simulink model "Q3b_state_space"  (R2025b)
settings: Solver=ode4  StartTime=0.0  StopTime=12.0  FixedStep=0.001  RelTol=1e-3
values from neighbouring files (symbols this model uses):
  A_aug = [A(1,1), A(1,2), 0, 0 ... (first row only)    [ME780_Part3b_Bicycle_DLC.m]
  B_aug = [B ... (first row only)    [ME780_Part3b_Bicycle_DLC.m]
  C_aug = [1,       0,          0, 0 ... (first row only)    [ME780_Part3b_Bicycle_DLC.m]
  D_aug = [0 ... (first row only)    [ME780_Part3b_Bicycle_DLC.m]
settings Model: Creator=r3anjum  LastModifiedBy=r3anjum

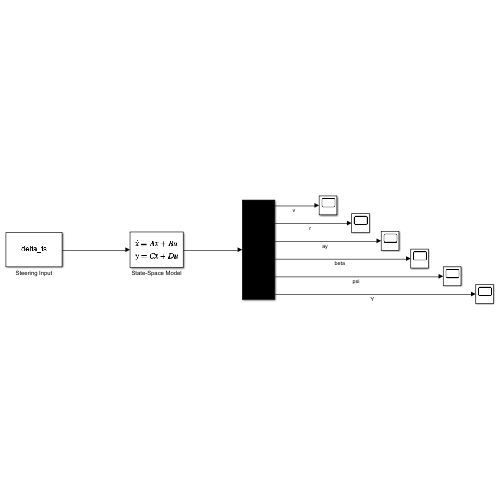
[thumbnail: Simulink's stored preview of the top-level diagram]
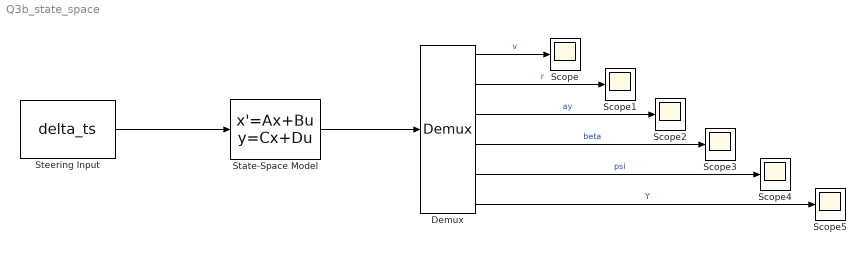
== system Q3b_state_space ==
  Demux : Demux  Outputs=6
  Scope{,1..5} (6 alike) : Scope
      Scope settings: ActiveDisplayYMinimum=-0.18345192277856021  ActiveDisplayYMaximum=0.18345192277856021
      Scope1 settings: ActiveDisplayYMinimum=-0.17826447483028088  ActiveDisplayYMaximum=0.17826447483028088
      Scope2 settings: ActiveDisplayYMinimum=-1.7516846511790012  ActiveDisplayYMaximum=1.7516846505365611  DataLoggingVariableName=ScopeData2
      Scope3 settings: ActiveDisplayYMinimum=-0.018869340628651907  ActiveDisplayYMaximum=0.018869340628651907  DataLoggingVariableName=ScopeData3
      Scope4 settings: ActiveDisplayYMinimum=-0.22734864104219266  ActiveDisplayYMaximum=0.22734864104219224  DataLoggingVariableName=ScopeData4
      Scope5 settings: ActiveDisplayYMinimum=-0.44354423507468116  ActiveDisplayYMaximum=3.9859160643032778  DataLoggingVariableName=ScopeData5
  State-Space Model : StateSpace  A=A_aug  B=B_aug  C=C_aug  D=D_aug  InitialCondition=[0; 0; 0; 0]
  Steering Input : FromWorkspace  VariableName=delta_ts
  wires:
  Steering Input/1 -> State-Space Model/1
  State-Space Model/1 -> Demux/1
  Demux/1 -> Scope/1  "v"
  Demux/2 -> Scope1/1  "r"
  Demux/3 -> Scope2/1  "ay"
  Demux/4 -> Scope3/1  "beta"
  Demux/5 -> Scope4/1  "psi"
  Demux/6 -> Scope5/1  "Y"
